simulink model "SIMULACION_RHONN_EFK"  (R2017b)
settings: Solver=VariableStepAuto  StartTime=0.0  StopTime=120  RelTol=1e-3
model workspace (MATLAB code in the model file):
  | %VALORES HUERISTICOS SEGUN EL PAPER
  | %NOTA : los valores cuya definicion se encuentre en minuscula
  | %se utiliza para generar de manera dinamica con programacion
  | %la variable final que se utiliza en el programa.
  | %De manera que si llegara a ser necesario solo se modificarian las variables iniciales
  | 
  | %VARIABLES INICIALES ========================================
  | 
  | p1 = 1 * (10^8);
  | p2 = 1 * (10^2);
  | p3 = 1 * (10^8);
  | p4 = 1 * (10^2);
  | p5 = 1 * (10^2);
  | p6 = 1 * (10^2);
  | p7 = 1 * (10^2);
  | 
  | r1 = 1 * (10^4);
  | r2 = 5 * (10^4);
  | r3 = 1 * (10^4);
  | r4 = 1 * (10^1);
  | r5 = 1 * (10^1);
  | r6 = 1 * (10^3);
  | r7 = 1 * (10^3);
  | 
  | q1 = 5 * (10^5);
  | q2 = 5 * (10^5);
  | q3 = 5 * (10^5);
  | q4 = 1 * (10^1);
  | q5 = 1 * (10^1);
  | q6 = 1 * (10^3);
  | q7 = 1 * (10^3);
  | 
  | G1 = 0.00001;
  | G2 = 0.00001;
  | 
  | %VALOREES INICIALES DE LOS PESOS USADOS EN EKF
  | 
  | %PESOS DE W1
  | W11 = 0.1;
  | W12 = 0.1;
  | %PESOS DE W2
  | W21 = 0.1;
  | W22 = 0.1;
  | %PESOS DE W3
  | W31 = 0.1;
  | W32 = 0.1;
  | %PESOS DE W4
  | W41 = 0.1;
  | W42 = 0.1;
  | W43 = 0.1;
  | W44 = 0.1;
  | %PESOS DE W5
  | W51 = 0.1;
  | W52 = 0.1;
  | W53 = 0.1;
  | W54 = 0.1;
  | %PESOS DE W6
  | W61 = 0.1;
  | W62 = 0.1;
  | W63 = 0.1;
  | W64 = 0.1;
  | %PESOS DE W7
  | W71 = 0.1;
  | W72 = 0.1;
  | W73 = 0.1;
  | W74 = 0.1;
  | 
  | %VALOR DE LAS SIGMOIDALES SUAVES
  | B = 2 * exp(-3);    %Este valor debe ser mayor a cero pero en base a mis observaciones menor a 1.
  | FO = 0.83;   %Este valor es obtenido de la tesis de la Dra Alma debe ser CERCANO y MENOR a 1, si este se vuelve 1 funcionara como FKE unicamente
  | 
  | 
  | %VARIABLES FINALES ========================================
  | 
  | %PARAMETROS DE ENTRENAMIENTO EKF PARA RHONN 1
  | W1 = [W11; W12]; %VALOR INICIAL de Vector de pesos para x1
  | P1 = diag([p1, p1]); %VALOR INICIAL de Matriz diagonal inicial de P1
  | R1 = r1; % Valor de R1
  | Q1 = diag([q1, q1]); % Valor de Q1
  | 
  | %PARAMETROS DE ENTRENAMIENTO EKF PARA RHONN 2
  | W2 = [W21; W22]; %VALOR INICIAL de Vector de pesos para x2
  | P2 = diag([p2, p2]); %VALOR INICIAL de Matriz diagonal inicial de P2
  | R2 = r2; % Valor de R2
  | Q2 = diag([q2, q2]); % Valor de Q2
  | 
  | %PARAMETROS DE ENTRENAMIENTO EKF PARA RHONN 3
  | W3 = [W31; W32]; %VALOR INICIAL de Vector de pesos para x3
  | P3 = diag([p3, p3]); %VALOR INICIAL de Matriz diagonal inicial de P3
  | R3 = r3; % Valor de R3
  | Q3 = diag([q3, q3]); % Valor de Q3
  | 
  | %PARAMETROS DE ENTRENAMIENTO EKF PARA RHONN 4
  | W4 = [W41; W42; W43; W44]; %VALOR INICIAL de Vector de pesos para x4
  | P4 = diag([p4, p4, p4, p4]); %VALOR INICIAL de Matriz diagonal inicial de P4
  | R4 = r4; % Valor de R4
  | Q4 = diag([q4, q4, q4, q4]); % Valor de Q4
  | 
  | %PARAMETROS DE ENTRENAMIENTO EKF PARA RHONN 5
  | W5 = [W51; W52; W53; W54]; %VALOR INICIAL de Vector de pesos para x5
  | P5 = diag([p5, p5, p5, p5]); %VALOR INICIAL de Matriz diagonal inicial de P5
  | R5 = r5; % Valor de R5
  | Q5 = diag([q5, q5, q5, q5]); % Valor de Q5
  | 
  | %PARAMETROS DE ENTRENAMIENTO EKF PARA RHONN 6
  | W6 = [W61; W62; W63; W64]; %VALOR INICIAL de Vector de pesos para x6
  | P6 = diag([p6, p6, p6, p6]); %VALOR INICIAL de Matriz diagonal inicial de P6
  | R6 = r6; % Valor de R6
  | Q6 = diag([q6, q6, q6, q6]); % Valor de Q6
  | 
  | %PARAMETROS DE ENTRENAMIENTO EKF PARA RHONN 7
  | W7 = [W71; W72; W73; W74]; %VALOR INICIAL de Vector de pesos para x7
  | P7 = diag([p7, p7, p7, p7]); %VALOR INICIAL de Matriz diagonal inicial de P7
  | R7 = r7; % Valor de R7
  | Q7 = diag([q7, q7, q7, q7]); % Valor de Q7
libraries: simulink x5
(part 1 of 2)
settings Model: Creator=52324  LastModifiedBy=52324

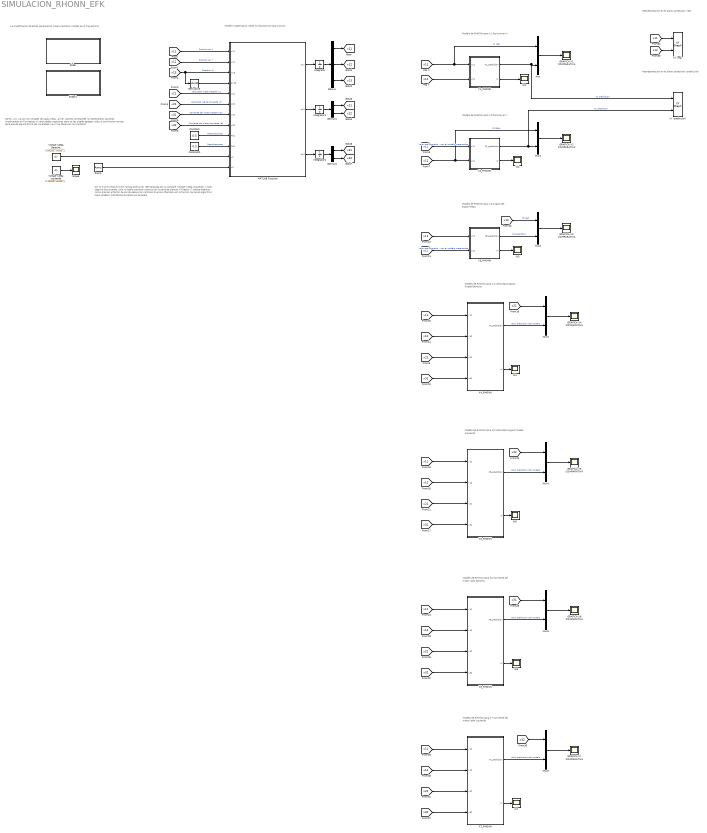
== system SIMULACION_RHONN_EFK ==
  note: por lo mismo esta funcion rampa podria ser reemplazada por la variable 'Voltaje rueda Izquierda'
      | y todo seguira funcionando, solo no habra cambios notorios en la serie de tiempo X4 hasta x7
      |
      | notese ademas como gracias al factor de olvido pese a los cambios bruscos ofrecidos por la funcion rampa
      | el algoritmo logra predecir satisfactoriamente sus estados.
  note: NOTA:
      | u1 y u2 son los voltajes de cada rueda ,
      | al ser valores constantes no representan cambios
      | importantes en Corriestes ni velocidades angulares
      | pero se les puede agregar ruido, o una funcion rampa
      | para que de alguna forma las varaiables x4-x7 se observen con cambios
  note: Representacion en el plano cartesiano 'real'
  note: La modificacion de estos parametros causa cambios visibles en la trayectoria
  note: Modelo matematico robot no holonomico tipo uniciclo
  note: Modelo de RHONN para X1
      | Posicion en X
  note: Modelo de RHONN para X2
      | Posicion en Y
  note: Modelo de RHONN para X3
      | Angulo del Robot Theta
  note: Modelo de RHONN para X4
      | Velocidad Angular Rueda Derecha
  note: Modelo de RHONN para X5
      | Velocidad Angular Rueda Izquierda
  note: Modelo de RHONN para X6
      | Corriente del motor lado derecho
  note: Modelo de RHONN para X7
      | Corriente del motor lado izquierdo
  note: Representacion en el plano cartesiano 'prediccion'
  Constant : Constant  Value=0.5
  Constant1 : Constant  Value=0.5
  Demux : Demux  Outputs=3
  Demux1 : Demux  Outputs=2
  Demux3 : Demux  Outputs=2
  Derivative : Derivative
  GRAFICA X1 COMPARATIVA : Scope
  GRAFICA X2 COMPARATIVA : Scope
  GRAFICA X3 COMPARATIVA : Scope
  GRAFICA X4 COMPARATIVA : Scope
  GRAFICA X5 COMPARATIVA : Scope
  GRAFICA X6 COMPARATIVA : Scope
  GRAFICA X7 COMPARATIVA : Scope
  Integrator : Integrator  InitialCondition=0.1
  Integrator1 : Integrator  InitialCondition=0.1
  Integrator2 : Integrator  InitialCondition=0.1
  MATLAB Function : MATLAB Function  TreatAsAtomicUnit=on
  Mux{,1..6} (7 alike) : Mux  Inputs=2
  Ramp : simulink/Sources/Ramp  slope=0.1  start=0  X0=0
  Scope : Scope
  Slider : Subsystem  DialogController=hmiCreateDDGDialog  IsWebBlock=on  mask(MWDashboardBlock){webBlockId=cf94a416-9279-4ce0-9e8d-8dce151b4ff8, webBlockType=slider, ShowInLibBrowser=on, ShowInitialText=on, HMISrcModelName=SIMULACION_RHONN_EFK}
      mask prompts: webBlockId "WebBlock Id"; webBlockType "WebBlock Type"; HMISrcModelName "Source Model"
      mask help: SimulinkHMI:dialogs:SliderDialogDesc
      mask Help: helpview([docroot '/mapfiles/simulink.map'], 'hmi_slider')
      mask Display:
      | if strcmp(get_param(bdroot(gcb),'BlockDiagramType'), 'library')
      |     image([(matlabroot) '/toolbox/simulink/hmi/icons/Slider.png']);
      | end
  Slider1 : Subsystem  DialogController=hmiCreateDDGDialog  IsWebBlock=on  mask(MWDashboardBlock){webBlockId=98018c70-82f4-44f7-8efb-1d66dbfb8826, webBlockType=slider, ShowInLibBrowser=on, ShowInitialText=on, HMISrcModelName=SIMULACION_RHONN_EFK}
      mask prompts: webBlockId "WebBlock Id"; webBlockType "WebBlock Type"; HMISrcModelName "Source Model"
      mask help: SimulinkHMI:dialogs:SliderDialogDesc
      mask Help: helpview([docroot '/mapfiles/simulink.map'], 'hmi_slider')
      mask Display:
      | if strcmp(get_param(bdroot(gcb),'BlockDiagramType'), 'library')
      |     image([(matlabroot) '/toolbox/simulink/hmi/icons/Slider.png']);
      | end
  Voltaje rueda Derecha : Constant  Value=0.6928571428571
  Voltaje rueda Izquierda : Constant  Value=0.1928571428571
  W{1..7} (7 alike) : Scope
  X1_RHONN : Subsystem
  X2_RHONN : Subsystem
  X3_RHONN : Subsystem
  X4_RHONN : Subsystem
  X5_RHONN : Subsystem
  X6_RHONN : Subsystem
  X7_RHONN : Subsystem
  XY 'prediccion' : simulink/Sinks/XY Graph  xmin=-2.5  xmax=2.5  ymin=-2.5  ymax=2.5  st=-1
  XY 'real' : simulink/Sinks/XY Graph  xmin=-2.5  xmax=2.5  ymin=-2.5  ymax=2.5  st=-1
  tag scope: x11=global, x12=global, x13=global, x21=global, x22=global, x31=global, x32=global
  wires:
  [x11] -> MATLAB Function/1(x11)  "Posicion en X"
  [x12] -> MATLAB Function/2(x12)  "Posicion en Y"
  MATLAB Function/1(dx1) -> Integrator/1
  [x13] -> Derivative/1, MATLAB Function/3(x13)  "Rotacion W"
  Derivative/1 -> MATLAB Function/4(dx13)
  Integrator/1 -> Demux/1
  Demux/3 -> [x13]
  Demux/2 -> [x12]
  MATLAB Function/2(dx2) -> Integrator1/1
  MATLAB Function/3(dx3) -> Integrator2/1
  Integrator1/1 -> Demux1/1
  Integrator2/1 -> Demux3/1
  [x21] -> MATLAB Function/5(x21)  "Velocidad rueda derecha V1"
  [x22] -> MATLAB Function/6(x22)  "Velocidad rueda izquierda V2"
  [x32] -> MATLAB Function/8(x32)  "Corriente del motor izquierdo Ia2"
  Demux1/1 -> [x21]
  Demux1/2 -> [x22]
  Demux3/1 -> [x31]
  Demux3/2 -> [x32]
  Constant/1 -> MATLAB Function/9(Td1)  "Perturbaciones"
  Constant1/1 -> MATLAB Function/10(Td2)  "Perturbaciones"
  X1_RHONN/1(X1_prediction) -> XY 'prediccion'/1, Mux/2  "X1 prediccion"
  Mux/1 -> GRAFICA X1 COMPARATIVA/1
  [x12] -> X1_RHONN/2(x12)
  [x11] -> Mux/1, X1_RHONN/1(x11)  "X1 real"
  [x12] -> Mux1/1, X2_RHONN/2(x12)  "X2 REAL"
  Mux1/1 -> GRAFICA X2 COMPARATIVA/1
  [x11] -> X2_RHONN/1(x11)  "Valor real arrojado por el modelo matematico"
  X2_RHONN/1(X2_prediction) -> XY 'prediccion'/2, Mux1/2  "X2 prediccion"
  [x11] -> X3_RHONN/1(x11)
  [x12] -> X3_RHONN/2(x12)  "Valor real arrojado por el modelo matematico"
  Mux2/1 -> GRAFICA X3 COMPARATIVA/1
  X3_RHONN/1(X3_prediction) -> Mux2/2  "X3 prediccion"
  [x21] -> Mux3/1
  Mux3/1 -> GRAFICA X4 COMPARATIVA/1
  [x12] -> X4_RHONN/2(x12)
  [x11] -> X4_RHONN/1(x11)
  X4_RHONN/1(X4_prediction) -> Mux3/2  "Valor prediccion del modelo"
  [x21] -> X4_RHONN/3(x21)
  [x31] -> X4_RHONN/4(x31)
  [x13] -> Mux2/1  "X3 real"
  [x11] -> X5_RHONN/1(x11)
  X5_RHONN/1(X5_prediction) -> Mux4/2  "Valor prediccion del modelo"
  [x22] -> Mux4/1
  [x12] -> X5_RHONN/2(x12)
  Mux4/1 -> GRAFICA X5 COMPARATIVA/1
  [x21] -> X5_RHONN/3(x21)
  [x31] -> X5_RHONN/4(x31)
  [x31] -> Mux5/1
  [x32] -> X6_RHONN/4(x32)
  [x22] -> X6_RHONN/3(x22)
  Mux5/1 -> GRAFICA X6 COMPARATIVA/1
  [x12] -> X6_RHONN/2(x12)
  X6_RHONN/1(X6_prediction) -> Mux5/2  "Valor prediccion del modelo"
  [x11] -> X6_RHONN/1(x11)
  [x32] -> X7_RHONN/4(x32)
  [x11] -> X7_RHONN/1(x11)
  Mux6/1 -> GRAFICA X7 COMPARATIVA/1
  [x22] -> X7_RHONN/3(x22)
  [x12] -> X7_RHONN/2(x12)
  X7_RHONN/1(X7_prediction) -> Mux6/2  "Valor prediccion del modelo"
  [x32] -> Mux6/1
  X1_RHONN/2(W) -> W1/1
  Demux/1 -> [x11]
  X2_RHONN/2(W) -> W2/1
  X3_RHONN/2(W) -> W3/1
  X4_RHONN/2(W) -> W4/1
  X5_RHONN/2(W) -> W5/1
  X6_RHONN/2(W) -> W6/1
  X7_RHONN/2(W) -> W7/1
  [x31] -> MATLAB Function/7(x31)  "Corriente del motor derecho Ia1"
  [x11] -> XY 'real'/1
  [x12] -> XY 'real'/2
  Voltaje rueda Derecha/1 -> MATLAB Function/11(u1)
  Ramp/1 -> MATLAB Function/12(u2)
  Voltaje rueda Izquierda/1 -> Scope/1

== system SIMULACION_RHONN_EFK/Slider ==

== system SIMULACION_RHONN_EFK/Slider1 ==

== system SIMULACION_RHONN_EFK/X1_RHONN ==
  note: Filtro extendido de kalman (EKF)
  note: Funcion RHONN
      |
      | X(k+1) = w11 * S(x11) + w12 * S(x12)
  x11 : Inport
  x12 : Inport  Port=2
  Generador de matriz H : MATLAB Function  TreatAsAtomicUnit=on
  Sigmoidal suave1 : Subsystem
  Sigmoidal suave3 : Subsystem
  X1_EKF : Subsystem
  X1_RHONN : MATLAB Function  TreatAsAtomicUnit=on
  X1_prediction : Outport
  W : Outport  Port=2
  wires:
  X1_RHONN/1(pred) -> X1_EKF/2(prediccion), X1_prediction/1  "Valor predicho por la red neuronal"
  Sigmoidal suave3/1(salida) -> Generador de matriz H/2(Sx12), X1_RHONN/3(Sx12)  "S(x12)"
  x12/1 -> Sigmoidal suave3/1(c)
  x11/1 -> X1_EKF/1(medicion), Sigmoidal suave1/1(c)
  Sigmoidal suave1/1(salida) -> Generador de matriz H/1(Sx11), X1_RHONN/2(Sx11)  "S(x11)"
  Generador de matriz H/1(H) -> X1_EKF/3(H)  "Valor de matriz H"
  X1_EKF/1(W) -> W/1, X1_RHONN/1(W)  "Valor actualizado de los pesos"

== system SIMULACION_RHONN_EFK/X2_RHONN ==
  note: Filtro extendido de kalman (EKF)
  note: Funcion RHONN
      |
      | X2(k+1) = w21 * S(x11) + w22 * S(x12)
  x11 : Inport
  x12 : Inport  Port=2
  Generador de matriz H : MATLAB Function  TreatAsAtomicUnit=on
  Sigmoidal suave1 : Subsystem
  Sigmoidal suave3 : Subsystem
  X2_EKF : Subsystem
  X2_RHONN_function : MATLAB Function  TreatAsAtomicUnit=on
  X2_prediction : Outport
  W : Outport  Port=2
  wires:
  X2_RHONN_function/1(pred) -> X2_EKF/2(prediccion), X2_prediction/1  "Valor predicho por la red neuronal"
  Sigmoidal suave3/1(salida) -> Generador de matriz H/2(Sx12), X2_RHONN_function/3(Sx12)  "S(x12)"
  x12/1 -> X2_EKF/1(medicion), Sigmoidal suave3/1(c)
  x11/1 -> Sigmoidal suave1/1(c)
  Sigmoidal suave1/1(salida) -> Generador de matriz H/1(Sx11), X2_RHONN_function/2(Sx11)  "S(x11)"
  Generador de matriz H/1(H) -> X2_EKF/3(H)  "Valor de matriz H"
  X2_EKF/1(W) -> X2_RHONN_function/1(W), W/1  "Valor actualizado de los pesos"

== system SIMULACION_RHONN_EFK/X3_RHONN ==
  note: Para este caso el error debe ser basado a la medicion del angulo del robot (x13)
  note: Filtro extendido de kalman (EKF)
  note: Funcion RHONN
      |
      | X3(k+1) = w31 * S(x11) + w32 * S(x12)
  x11 : Inport
  x12 : Inport  Port=2
  Generador de matriz H : MATLAB Function  TreatAsAtomicUnit=on
  Sigmoidal suave1 : Subsystem
  Sigmoidal suave3 : Subsystem
  X3_EKF : Subsystem
  X3_RHONN_function : MATLAB Function  TreatAsAtomicUnit=on
  X3_prediction : Outport
  W : Outport  Port=2
  wires:
  X3_RHONN_function/1(pred) -> X3_EKF/2(prediccion), X3_prediction/1  "Valor predicho por la red neuronal"
  Sigmoidal suave3/1(salida) -> Generador de matriz H/2(Sx12), X3_RHONN_function/3(Sx12)  "S(x12)"
  x12/1 -> Sigmoidal suave3/1(c)
  x11/1 -> Sigmoidal suave1/1(c)
  Sigmoidal suave1/1(salida) -> Generador de matriz H/1(Sx11), X3_RHONN_function/2(Sx11)  "S(x11)"
  Generador de matriz H/1(H) -> X3_EKF/3(H)  "Valor de matriz H"
  X3_EKF/1(W) -> W/1, X3_RHONN_function/1(W)  "Valor actualizado de los pesos"
  [x13] -> X3_EKF/1(medicion)  "Angulo del robot medido"

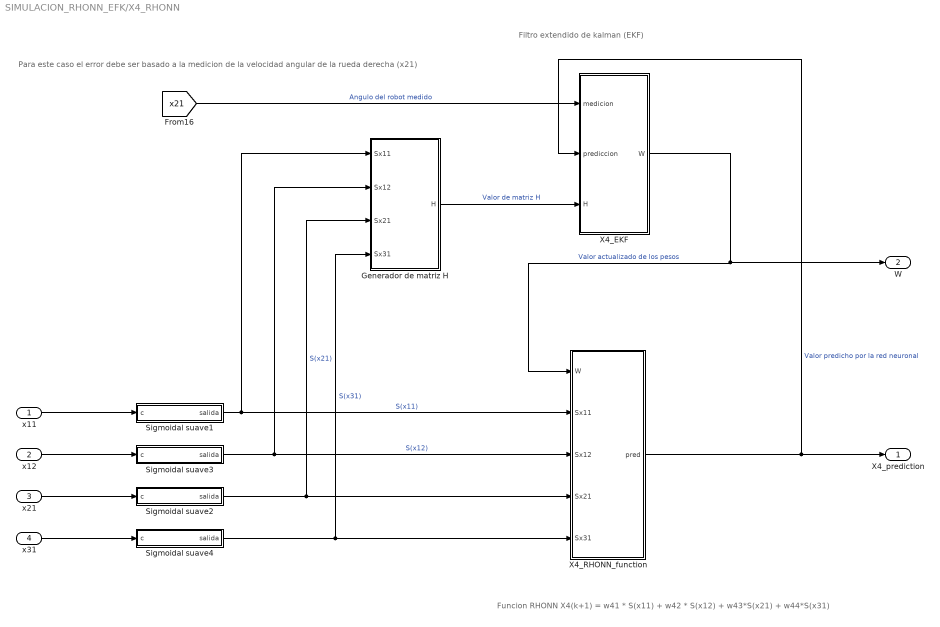
== system SIMULACION_RHONN_EFK/X4_RHONN ==
  note: Para este caso el error debe ser basado a la medicion de la velocidad angular de la rueda derecha (x21)
  note: Filtro extendido de kalman (EKF)
  note: Funcion RHONN
      |
      | X4(k+1) = w41 * S(x11) + w42 * S(x12) + w43*S(x21) + w44*S(x31)
  x11 : Inport
  x12 : Inport  Port=2
  x21 : Inport  Port=3
  x31 : Inport  Port=4
  Generador de matriz H : MATLAB Function  TreatAsAtomicUnit=on
  Sigmoidal suave1 : Subsystem
  Sigmoidal suave2 : Subsystem
  Sigmoidal suave3 : Subsystem
  Sigmoidal suave4 : Subsystem
  X4_EKF : Subsystem
  X4_RHONN_function : MATLAB Function  TreatAsAtomicUnit=on
  X4_prediction : Outport
  W : Outport  Port=2
  wires:
  X4_RHONN_function/1(pred) -> X4_EKF/2(prediccion), X4_prediction/1  "Valor predicho por la red neuronal"
  Sigmoidal suave3/1(salida) -> Generador de matriz H/2(Sx12), X4_RHONN_function/3(Sx12)  "S(x12)"
  x12/1 -> Sigmoidal suave3/1(c)
  x11/1 -> Sigmoidal suave1/1(c)
  Sigmoidal suave1/1(salida) -> Generador de matriz H/1(Sx11), X4_RHONN_function/2(Sx11)  "S(x11)"
  Generador de matriz H/1(H) -> X4_EKF/3(H)  "Valor de matriz H"
  X4_EKF/1(W) -> X4_RHONN_function/1(W), W/1  "Valor actualizado de los pesos"
  [x21] -> X4_EKF/1(medicion)  "Angulo del robot medido"
  x21/1 -> Sigmoidal suave2/1(c)
  x31/1 -> Sigmoidal suave4/1(c)
  Sigmoidal suave2/1(salida) -> Generador de matriz H/3(Sx21), X4_RHONN_function/4(Sx21)  "S(x21)"
  Sigmoidal suave4/1(salida) -> Generador de matriz H/4(Sx31), X4_RHONN_function/5(Sx31)  "S(x31)"

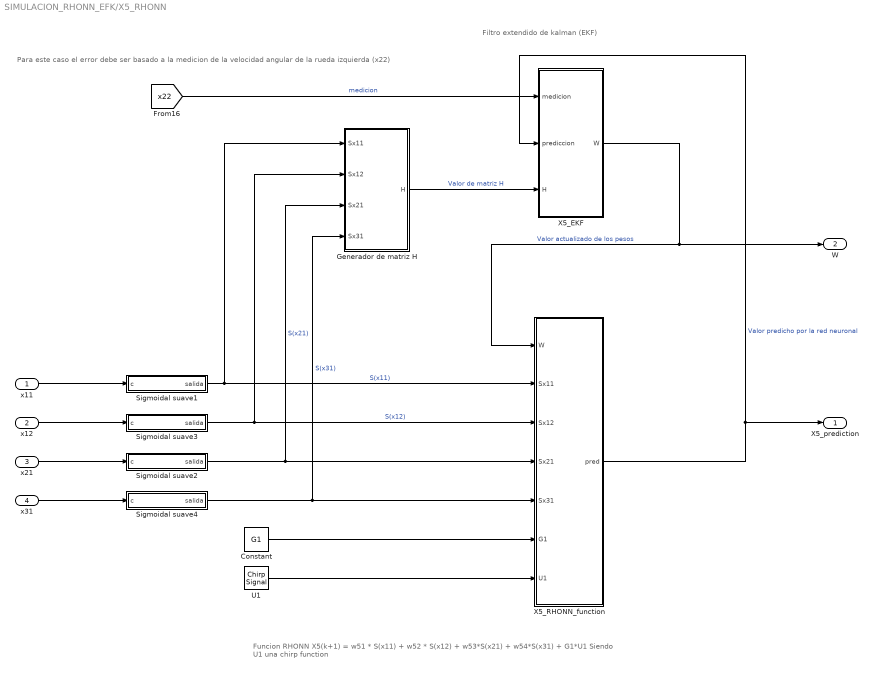
== system SIMULACION_RHONN_EFK/X5_RHONN ==
  note: Para este caso el error debe ser basado a la medicion de la velocidad angular de la rueda izquierda (x22)
  note: Filtro extendido de kalman (EKF)
  note: Funcion RHONN
      |
      | X5(k+1) = w51 * S(x11) + w52 * S(x12) + w53*S(x21) + w54*S(x31) + G1*U1
      |
      | Siendo U1 una chirp function
  x11 : Inport
  x12 : Inport  Port=2
  x21 : Inport  Port=3
  x31 : Inport  Port=4
  Constant : Constant  Value=G1
  Generador de matriz H : MATLAB Function  TreatAsAtomicUnit=on
  Sigmoidal suave1 : Subsystem
  Sigmoidal suave2 : Subsystem
  Sigmoidal suave3 : Subsystem
  Sigmoidal suave4 : Subsystem
  U1 : simulink/Sources/Chirp Signal  f1=0.1  T=100  f2=1
  X5_EKF : Subsystem
  X5_RHONN_function : MATLAB Function  TreatAsAtomicUnit=on
  X5_prediction : Outport
  W : Outport  Port=2
  wires:
  X5_RHONN_function/1(pred) -> X5_EKF/2(prediccion), X5_prediction/1  "Valor predicho por la red neuronal"
  Sigmoidal suave3/1(salida) -> Generador de matriz H/2(Sx12), X5_RHONN_function/3(Sx12)  "S(x12)"
  x12/1 -> Sigmoidal suave3/1(c)
  x11/1 -> Sigmoidal suave1/1(c)
  Sigmoidal suave1/1(salida) -> Generador de matriz H/1(Sx11), X5_RHONN_function/2(Sx11)  "S(x11)"
  Generador de matriz H/1(H) -> X5_EKF/3(H)  "Valor de matriz H"
  X5_EKF/1(W) -> W/1, X5_RHONN_function/1(W)  "Valor actualizado de los pesos"
  [x22] -> X5_EKF/1(medicion)  "medicion"
  x21/1 -> Sigmoidal suave2/1(c)
  x31/1 -> Sigmoidal suave4/1(c)
  Sigmoidal suave2/1(salida) -> Generador de matriz H/3(Sx21), X5_RHONN_function/4(Sx21)  "S(x21)"
  Sigmoidal suave4/1(salida) -> Generador de matriz H/4(Sx31), X5_RHONN_function/5(Sx31)  "S(x31)"
  Constant/1 -> X5_RHONN_function/6(G1)
  U1/1 -> X5_RHONN_function/7(U1)

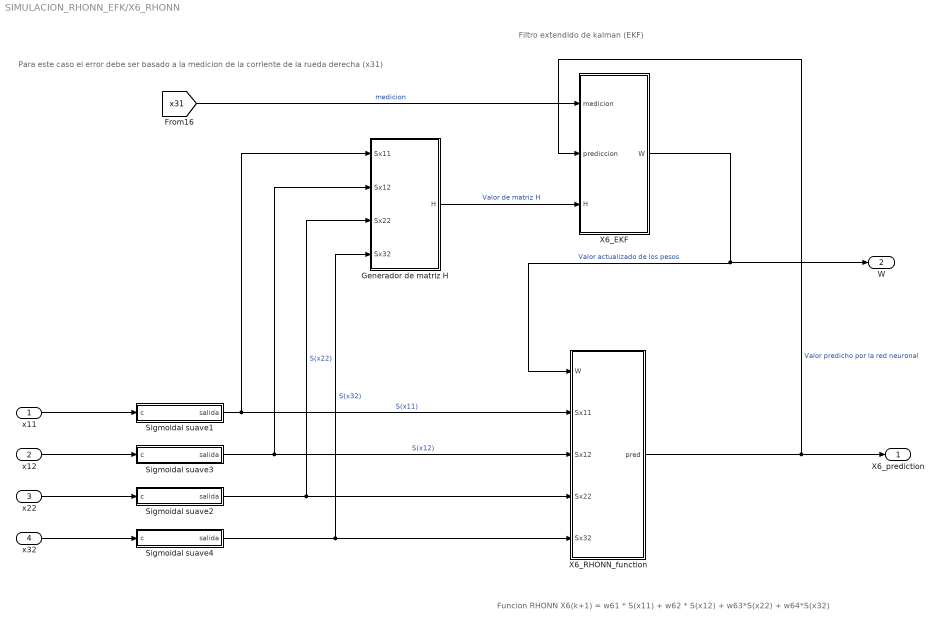
== system SIMULACION_RHONN_EFK/X6_RHONN ==
  note: Para este caso el error debe ser basado a la medicion de la corriente de la rueda derecha (x31)
  note: Filtro extendido de kalman (EKF)
  note: Funcion RHONN
      |
      | X6(k+1) = w61 * S(x11) + w62 * S(x12) + w63*S(x22) + w64*S(x32)
  x11 : Inport
  x12 : Inport  Port=2
  x22 : Inport  Port=3
  x32 : Inport  Port=4
  Generador de matriz H : MATLAB Function  TreatAsAtomicUnit=on
  Sigmoidal suave1 : Subsystem
  Sigmoidal suave2 : Subsystem
  Sigmoidal suave3 : Subsystem
  Sigmoidal suave4 : Subsystem
  X6_EKF : Subsystem
  X6_RHONN_function : MATLAB Function  TreatAsAtomicUnit=on
  X6_prediction : Outport
  W : Outport  Port=2
  wires:
  X6_RHONN_function/1(pred) -> X6_EKF/2(prediccion), X6_prediction/1  "Valor predicho por la red neuronal"
  Sigmoidal suave3/1(salida) -> Generador de matriz H/2(Sx12), X6_RHONN_function/3(Sx12)  "S(x12)"
  x12/1 -> Sigmoidal suave3/1(c)
  x11/1 -> Sigmoidal suave1/1(c)
  Sigmoidal suave1/1(salida) -> Generador de matriz H/1(Sx11), X6_RHONN_function/2(Sx11)  "S(x11)"
  Generador de matriz H/1(H) -> X6_EKF/3(H)  "Valor de matriz H"
  X6_EKF/1(W) -> W/1, X6_RHONN_function/1(W)  "Valor actualizado de los pesos"
  [x31] -> X6_EKF/1(medicion)  "medicion"
  x22/1 -> Sigmoidal suave2/1(c)
  x32/1 -> Sigmoidal suave4/1(c)
  Sigmoidal suave2/1(salida) -> Generador de matriz H/3(Sx22), X6_RHONN_function/4(Sx22)  "S(x22)"
  Sigmoidal suave4/1(salida) -> Generador de matriz H/4(Sx32), X6_RHONN_function/5(Sx32)  "S(x32)"

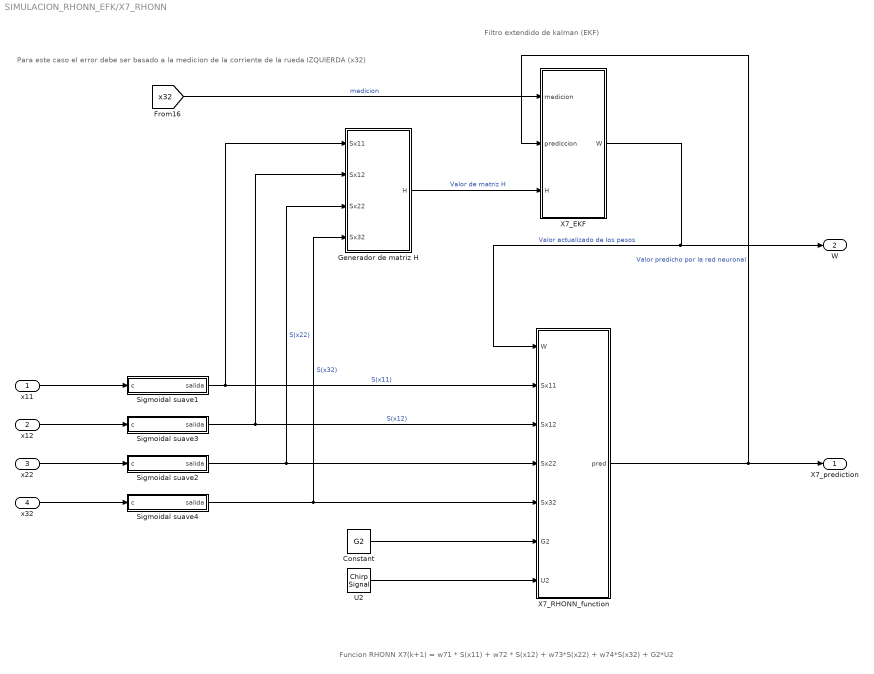
== system SIMULACION_RHONN_EFK/X7_RHONN ==
  note: Para este caso el error debe ser basado a la medicion de la corriente de la rueda IZQUIERDA (x32)
  note: Filtro extendido de kalman (EKF)
  note: Funcion RHONN
      |
      | X7(k+1) = w71 * S(x11) + w72 * S(x12) + w73*S(x22) + w74*S(x32) + G2*U2
  x11 : Inport
  x12 : Inport  Port=2
  x22 : Inport  Port=3
  x32 : Inport  Port=4
  Constant : Constant  Value=G2
  Generador de matriz H : MATLAB Function  TreatAsAtomicUnit=on
  Sigmoidal suave1 : Subsystem
  Sigmoidal suave2 : Subsystem
  Sigmoidal suave3 : Subsystem
  Sigmoidal suave4 : Subsystem
  U2 : simulink/Sources/Chirp Signal  f1=0.1  T=100  f2=1
  X7_EKF : Subsystem
  X7_RHONN_function : MATLAB Function  TreatAsAtomicUnit=on
  X7_prediction : Outport
  W : Outport  Port=2
  wires:
  X7_RHONN_function/1(pred) -> X7_EKF/2(prediccion), X7_prediction/1  "Valor predicho por la red neuronal"
  Sigmoidal suave3/1(salida) -> Generador de matriz H/2(Sx12), X7_RHONN_function/3(Sx12)  "S(x12)"
  x12/1 -> Sigmoidal suave3/1(c)
  x11/1 -> Sigmoidal suave1/1(c)
  Sigmoidal suave1/1(salida) -> Generador de matriz H/1(Sx11), X7_RHONN_function/2(Sx11)  "S(x11)"
  Generador de matriz H/1(H) -> X7_EKF/3(H)  "Valor de matriz H"
  X7_EKF/1(W) -> W/1, X7_RHONN_function/1(W)  "Valor actualizado de los pesos"
  [x32] -> X7_EKF/1(medicion)  "medicion"
  x22/1 -> Sigmoidal suave2/1(c)
  x32/1 -> Sigmoidal suave4/1(c)
  Sigmoidal suave2/1(salida) -> Generador de matriz H/3(Sx22), X7_RHONN_function/4(Sx22)  "S(x22)"
  Sigmoidal suave4/1(salida) -> Generador de matriz H/4(Sx32), X7_RHONN_function/5(Sx32)  "S(x32)"
  Constant/1 -> X7_RHONN_function/6(G2)
  U2/1 -> X7_RHONN_function/7(U2)

== system SIMULACION_RHONN_EFK/X1_RHONN/Sigmoidal suave1 ==
  note: Funcion sigmoidal suave S(*)
  note: Dada la ecuacion (5) del paper:
      | B > 0
      |
      | Y observado en la tesis de la Dra Alma
      | B = 2e^-3
  c : Inport
  Constante de sigmoidal suave : Constant  Value=B
  Sigmoidal suave : MATLAB Function  TreatAsAtomicUnit=on
  salida : Outport
  wires:
  Sigmoidal suave/1(sig) -> salida/1  "Señal transformada S(*)"
  c/1 -> Sigmoidal suave/2(c)  "Señal a transformar"
  Constante de sigmoidal suave/1 -> Sigmoidal suave/1(B)

== system SIMULACION_RHONN_EFK/X1_RHONN/Sigmoidal suave3 ==
  note: Funcion sigmoidal suave S(*)
  note: Dada la ecuacion (5) del paper:
      | B > 0
      |
      | Y observado en la tesis de la Dra Alma
      | B = 2e^-3
  c : Inport
  Constante de sigmoidal suave : Constant  Value=B
  Sigmoidal suave : MATLAB Function  TreatAsAtomicUnit=on
  salida : Outport
  wires:
  Sigmoidal suave/1(sig) -> salida/1  "Señal transformada S(*)"
  c/1 -> Sigmoidal suave/2(c)  "Señal a transformar"
  Constante de sigmoidal suave/1 -> Sigmoidal suave/1(B)

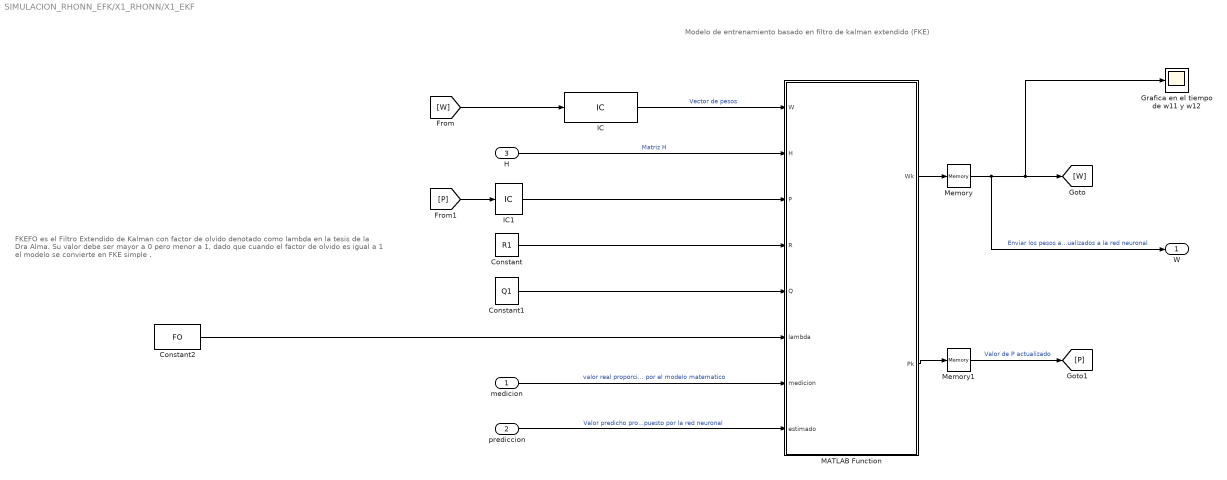
== system SIMULACION_RHONN_EFK/X1_RHONN/X1_EKF ==
  note: FKEFO es el Filtro Extendido de Kalman con factor de olvido
      |
      | denotado como lambda en la tesis de la Dra Alma.
      | Su valor debe ser mayor a 0 pero menor a 1, dado que cuando
      | el factor de olvido es igual a 1 el modelo se convierte en FKE simple .
  note: Modelo de entrenamiento basado en filtro de kalman extendido (FKE)
  medicion : Inport
  prediccion : Inport  Port=2
  H : Inport  Port=3
  Constant : Constant  Value=R1
  Constant1 : Constant  Value=Q1
  Constant2 : Constant  Value=FO
  Grafica en el tiempo de w11 y w12 : Scope
  IC : InitialCondition  Value=W1
  IC1 : InitialCondition  Value=P1
  MATLAB Function : MATLAB Function  TreatAsAtomicUnit=on
  Memory : Memory
  Memory1 : Memory
  W : Outport
  wires:
  prediccion/1 -> MATLAB Function/8(estimado)  "Valor predicho propuesto por la red neuronal"
  medicion/1 -> MATLAB Function/7(medicion)  "valor real proporcionado por el modelo matematico"
  MATLAB Function/1(Wk) -> Memory/1
  [W] -> IC/1
  IC/1 -> MATLAB Function/1(W)  "Vector de pesos"
  MATLAB Function/2(Pk) -> Memory1/1
  IC1/1 -> MATLAB Function/3(P)
  [P] -> IC1/1
  Constant/1 -> MATLAB Function/4(R)
  Constant1/1 -> MATLAB Function/5(Q)
  H/1 -> MATLAB Function/2(H)  "Matriz H"
  Memory1/1 -> [P]  "Valor de P actualizado"
  Memory/1 -> Grafica en el tiempo de w11 y w12/1, [W], W/1  "Enviar los pesos actualizados a la red neuronal"
  Constant2/1 -> MATLAB Function/6(lambda)

== system SIMULACION_RHONN_EFK/X2_RHONN/Sigmoidal suave1 ==
  note: Funcion sigmoidal suave S(*)
  note: Dada la ecuacion (5) del paper:
      | B > 0
      |
      | Y observado en la tesis de la Dra Alma
      | B = 2e^-3
  c : Inport
  Constante de sigmoidal suave : Constant  Value=B
  Sigmoidal suave : MATLAB Function  TreatAsAtomicUnit=on
  salida : Outport
  wires:
  Sigmoidal suave/1(sig) -> salida/1  "Señal transformada S(*)"
  c/1 -> Sigmoidal suave/2(c)  "Señal a transformar"
  Constante de sigmoidal suave/1 -> Sigmoidal suave/1(B)

== system SIMULACION_RHONN_EFK/X2_RHONN/Sigmoidal suave3 ==
  note: Funcion sigmoidal suave S(*)
  note: Dada la ecuacion (5) del paper:
      | B > 0
      |
      | Y observado en la tesis de la Dra Alma
      | B = 2e^-3
  c : Inport
  Constante de sigmoidal suave : Constant  Value=B
  Sigmoidal suave : MATLAB Function  TreatAsAtomicUnit=on
  salida : Outport
  wires:
  Sigmoidal suave/1(sig) -> salida/1  "Señal transformada S(*)"
  c/1 -> Sigmoidal suave/2(c)  "Señal a transformar"
  Constante de sigmoidal suave/1 -> Sigmoidal suave/1(B)

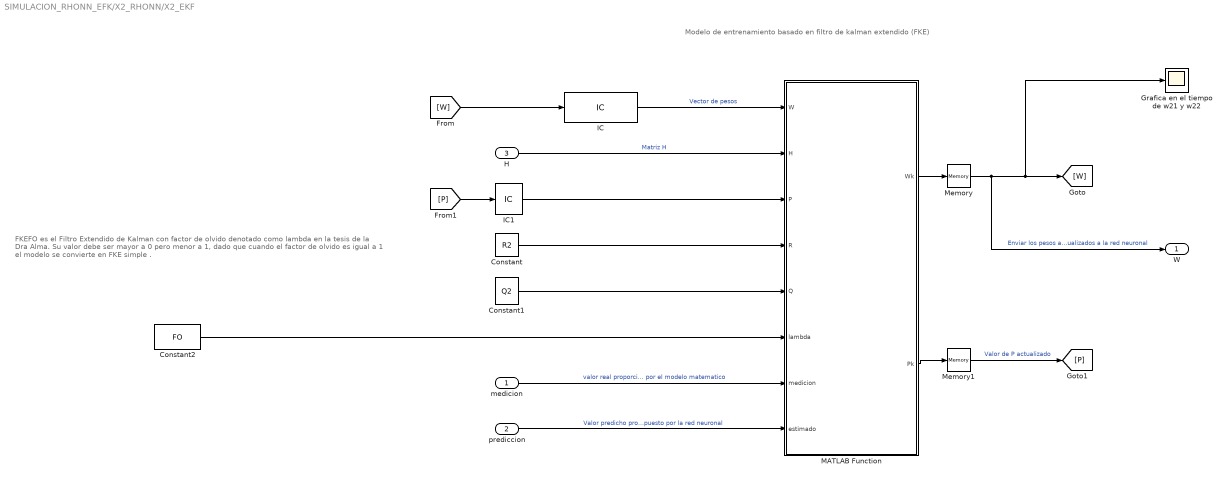
== system SIMULACION_RHONN_EFK/X2_RHONN/X2_EKF ==
  note: FKEFO es el Filtro Extendido de Kalman con factor de olvido
      |
      | denotado como lambda en la tesis de la Dra Alma.
      | Su valor debe ser mayor a 0 pero menor a 1, dado que cuando
      | el factor de olvido es igual a 1 el modelo se convierte en FKE simple .
  note: Modelo de entrenamiento basado en filtro de kalman extendido (FKE)
  medicion : Inport
  prediccion : Inport  Port=2
  H : Inport  Port=3
  Constant : Constant  Value=R2
  Constant1 : Constant  Value=Q2
  Constant2 : Constant  Value=FO
  Grafica en el tiempo de w21 y w22 : Scope
  IC : InitialCondition  Value=W2
  IC1 : InitialCondition  Value=P2
  MATLAB Function : MATLAB Function  TreatAsAtomicUnit=on
  Memory : Memory
  Memory1 : Memory
  W : Outport
  wires:
  prediccion/1 -> MATLAB Function/8(estimado)  "Valor predicho propuesto por la red neuronal"
  medicion/1 -> MATLAB Function/7(medicion)  "valor real proporcionado por el modelo matematico"
  MATLAB Function/1(Wk) -> Memory/1
  [W] -> IC/1
  IC/1 -> MATLAB Function/1(W)  "Vector de pesos"
  MATLAB Function/2(Pk) -> Memory1/1
  IC1/1 -> MATLAB Function/3(P)
  [P] -> IC1/1
  Constant/1 -> MATLAB Function/4(R)
  Constant1/1 -> MATLAB Function/5(Q)
  H/1 -> MATLAB Function/2(H)  "Matriz H"
  Memory1/1 -> [P]  "Valor de P actualizado"
  Memory/1 -> Grafica en el tiempo de w21 y w22/1, [W], W/1  "Enviar los pesos actualizados a la red neuronal"
  Constant2/1 -> MATLAB Function/6(lambda)

== system SIMULACION_RHONN_EFK/X3_RHONN/Sigmoidal suave1 ==
  note: Funcion sigmoidal suave S(*)
  note: Dada la ecuacion (5) del paper:
      | B > 0
      |
      | Y observado en la tesis de la Dra Alma
      | B = 2e^-3
  c : Inport
  Constante de sigmoidal suave : Constant  Value=B
  Sigmoidal suave : MATLAB Function  TreatAsAtomicUnit=on
  salida : Outport
  wires:
  Sigmoidal suave/1(sig) -> salida/1  "Señal transformada S(*)"
  c/1 -> Sigmoidal suave/2(c)  "Señal a transformar"
  Constante de sigmoidal suave/1 -> Sigmoidal suave/1(B)

== system SIMULACION_RHONN_EFK/X3_RHONN/Sigmoidal suave3 ==
  note: Funcion sigmoidal suave S(*)
  note: Dada la ecuacion (5) del paper:
      | B > 0
      |
      | Y observado en la tesis de la Dra Alma
      | B = 2e^-3
  c : Inport
  Constante de sigmoidal suave : Constant  Value=B
  Sigmoidal suave : MATLAB Function  TreatAsAtomicUnit=on
  salida : Outport
  wires:
  Sigmoidal suave/1(sig) -> salida/1  "Señal transformada S(*)"
  c/1 -> Sigmoidal suave/2(c)  "Señal a transformar"
  Constante de sigmoidal suave/1 -> Sigmoidal suave/1(B)

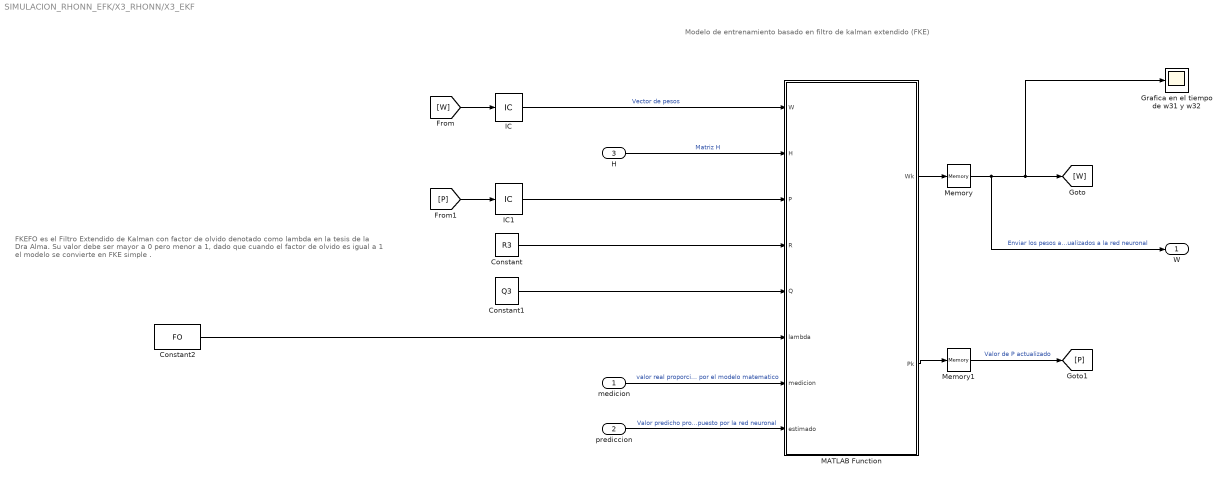
== system SIMULACION_RHONN_EFK/X3_RHONN/X3_EKF ==
  note: FKEFO es el Filtro Extendido de Kalman con factor de olvido
      |
      | denotado como lambda en la tesis de la Dra Alma.
      | Su valor debe ser mayor a 0 pero menor a 1, dado que cuando
      | el factor de olvido es igual a 1 el modelo se convierte en FKE simple .
  note: Modelo de entrenamiento basado en filtro de kalman extendido (FKE)
  medicion : Inport
  prediccion : Inport  Port=2
  H : Inport  Port=3
  Constant : Constant  Value=R3
  Constant1 : Constant  Value=Q3
  Constant2 : Constant  Value=FO
  Grafica en el tiempo de w31 y w32 : Scope
  IC : InitialCondition  Value=W3
  IC1 : InitialCondition  Value=P3
  MATLAB Function : MATLAB Function  TreatAsAtomicUnit=on
  Memory : Memory
  Memory1 : Memory
  W : Outport
  wires:
  prediccion/1 -> MATLAB Function/8(estimado)  "Valor predicho propuesto por la red neuronal"
  medicion/1 -> MATLAB Function/7(medicion)  "valor real proporcionado por el modelo matematico"
  MATLAB Function/1(Wk) -> Memory/1
  [W] -> IC/1
  IC/1 -> MATLAB Function/1(W)  "Vector de pesos"
  MATLAB Function/2(Pk) -> Memory1/1
  IC1/1 -> MATLAB Function/3(P)
  [P] -> IC1/1
  Constant/1 -> MATLAB Function/4(R)
  Constant1/1 -> MATLAB Function/5(Q)
  H/1 -> MATLAB Function/2(H)  "Matriz H"
  Memory1/1 -> [P]  "Valor de P actualizado"
  Memory/1 -> Grafica en el tiempo de w31 y w32/1, [W], W/1  "Enviar los pesos actualizados a la red neuronal"
  Constant2/1 -> MATLAB Function/6(lambda)

== system SIMULACION_RHONN_EFK/X4_RHONN/Sigmoidal suave1 ==
  note: Funcion sigmoidal suave S(*)
  note: Dada la ecuacion (5) del paper:
      | B > 0
      |
      | Y observado en la tesis de la Dra Alma
      | B = 2e^-3
  c : Inport
  Constante de sigmoidal suave : Constant  Value=B
  Sigmoidal suave : MATLAB Function  TreatAsAtomicUnit=on
  salida : Outport
  wires:
  Sigmoidal suave/1(sig) -> salida/1  "Señal transformada S(*)"
  c/1 -> Sigmoidal suave/2(c)  "Señal a transformar"
  Constante de sigmoidal suave/1 -> Sigmoidal suave/1(B)

== system SIMULACION_RHONN_EFK/X4_RHONN/Sigmoidal suave2 ==
  note: Funcion sigmoidal suave S(*)
  note: Dada la ecuacion (5) del paper:
      | B > 0
      |
      | Y observado en la tesis de la Dra Alma
      | B = 2e^-3
  c : Inport
  Constante de sigmoidal suave : Constant  Value=B
  Sigmoidal suave : MATLAB Function  TreatAsAtomicUnit=on
  salida : Outport
  wires:
  Sigmoidal suave/1(sig) -> salida/1  "Señal transformada S(*)"
  c/1 -> Sigmoidal suave/2(c)  "Señal a transformar"
  Constante de sigmoidal suave/1 -> Sigmoidal suave/1(B)

== system SIMULACION_RHONN_EFK/X4_RHONN/Sigmoidal suave3 ==
  note: Funcion sigmoidal suave S(*)
  note: Dada la ecuacion (5) del paper:
      | B > 0
      |
      | Y observado en la tesis de la Dra Alma
      | B = 2e^-3
  c : Inport
  Constante de sigmoidal suave : Constant  Value=B
  Sigmoidal suave : MATLAB Function  TreatAsAtomicUnit=on
  salida : Outport
  wires:
  Sigmoidal suave/1(sig) -> salida/1  "Señal transformada S(*)"
  c/1 -> Sigmoidal suave/2(c)  "Señal a transformar"
  Constante de sigmoidal suave/1 -> Sigmoidal suave/1(B)

== system SIMULACION_RHONN_EFK/X4_RHONN/Sigmoidal suave4 ==
  note: Funcion sigmoidal suave S(*)
  note: Dada la ecuacion (5) del paper:
      | B > 0
      |
      | Y observado en la tesis de la Dra Alma
      | B = 2e^-3
  c : Inport
  Constante de sigmoidal suave : Constant  Value=B
  Sigmoidal suave : MATLAB Function  TreatAsAtomicUnit=on
  salida : Outport
  wires:
  Sigmoidal suave/1(sig) -> salida/1  "Señal transformada S(*)"
  c/1 -> Sigmoidal suave/2(c)  "Señal a transformar"
  Constante de sigmoidal suave/1 -> Sigmoidal suave/1(B)

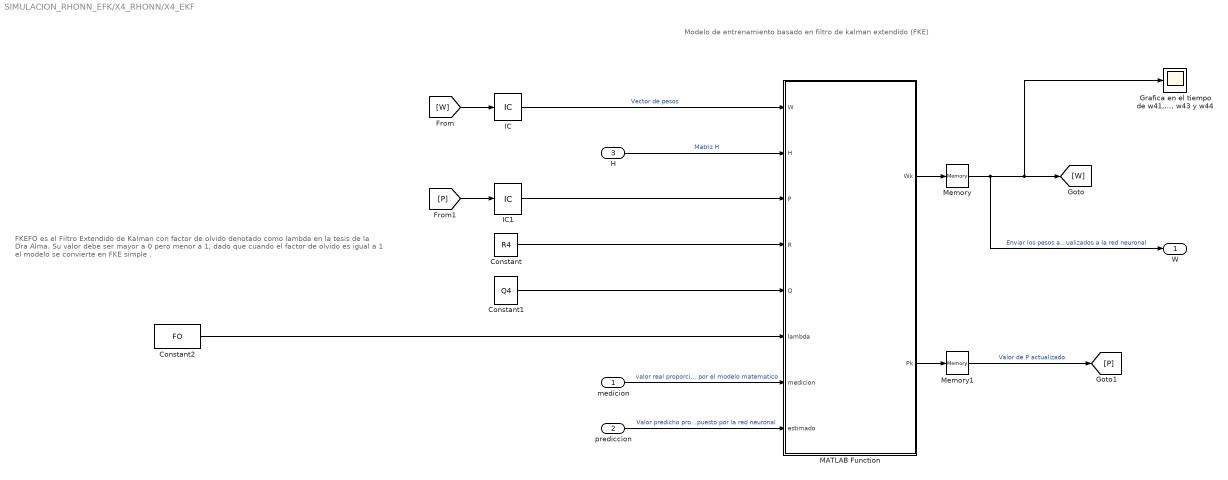
== system SIMULACION_RHONN_EFK/X4_RHONN/X4_EKF ==
  note: FKEFO es el Filtro Extendido de Kalman con factor de olvido
      |
      | denotado como lambda en la tesis de la Dra Alma.
      | Su valor debe ser mayor a 0 pero menor a 1, dado que cuando
      | el factor de olvido es igual a 1 el modelo se convierte en FKE simple .
  note: Modelo de entrenamiento basado en filtro de kalman extendido (FKE)
  medicion : Inport
  prediccion : Inport  Port=2
  H : Inport  Port=3
  Constant : Constant  Value=R4
  Constant1 : Constant  Value=Q4
  Constant2 : Constant  Value=FO
  "Grafica en el tiempo de w41, w42, w43 y w44" : Scope
  IC : InitialCondition  Value=W4
  IC1 : InitialCondition  Value=P4
  MATLAB Function : MATLAB Function  TreatAsAtomicUnit=on
  Memory : Memory
  Memory1 : Memory
  W : Outport
  wires:
  prediccion/1 -> MATLAB Function/8(estimado)  "Valor predicho propuesto por la red neuronal"
  medicion/1 -> MATLAB Function/7(medicion)  "valor real proporcionado por el modelo matematico"
  MATLAB Function/1(Wk) -> Memory/1
  [W] -> IC/1
  IC/1 -> MATLAB Function/1(W)  "Vector de pesos"
  MATLAB Function/2(Pk) -> Memory1/1
  IC1/1 -> MATLAB Function/3(P)
  [P] -> IC1/1
  Constant/1 -> MATLAB Function/4(R)
  Constant1/1 -> MATLAB Function/5(Q)
  H/1 -> MATLAB Function/2(H)  "Matriz H"
  Memory1/1 -> [P]  "Valor de P actualizado"
  Memory/1 -> "Grafica en el tiempo de w41, w42, w43 y w44"/1, [W], W/1  "Enviar los pesos actualizados a la red neuronal"
  Constant2/1 -> MATLAB Function/6(lambda)

== system SIMULACION_RHONN_EFK/X5_RHONN/Sigmoidal suave1 ==
  note: Funcion sigmoidal suave S(*)
  note: Dada la ecuacion (5) del paper:
      | B > 0
      |
      | Y observado en la tesis de la Dra Alma
      | B = 2e^-3
  c : Inport
  Constante de sigmoidal suave : Constant  Value=B
  Sigmoidal suave : MATLAB Function  TreatAsAtomicUnit=on
  salida : Outport
  wires:
  Sigmoidal suave/1(sig) -> salida/1  "Señal transformada S(*)"
  c/1 -> Sigmoidal suave/2(c)  "Señal a transformar"
  Constante de sigmoidal suave/1 -> Sigmoidal suave/1(B)

== system SIMULACION_RHONN_EFK/X5_RHONN/Sigmoidal suave2 ==
  note: Funcion sigmoidal suave S(*)
  note: Dada la ecuacion (5) del paper:
      | B > 0
      |
      | Y observado en la tesis de la Dra Alma
      | B = 2e^-3
  c : Inport
  Constante de sigmoidal suave : Constant  Value=B
  Sigmoidal suave : MATLAB Function  TreatAsAtomicUnit=on
  salida : Outport
  wires:
  Sigmoidal suave/1(sig) -> salida/1  "Señal transformada S(*)"
  c/1 -> Sigmoidal suave/2(c)  "Señal a transformar"
  Constante de sigmoidal suave/1 -> Sigmoidal suave/1(B)

== system SIMULACION_RHONN_EFK/X5_RHONN/Sigmoidal suave3 ==
  note: Funcion sigmoidal suave S(*)
  note: Dada la ecuacion (5) del paper:
      | B > 0
      |
      | Y observado en la tesis de la Dra Alma
      | B = 2e^-3
  c : Inport
  Constante de sigmoidal suave : Constant  Value=B
  Sigmoidal suave : MATLAB Function  TreatAsAtomicUnit=on
  salida : Outport
  wires:
  Sigmoidal suave/1(sig) -> salida/1  "Señal transformada S(*)"
  c/1 -> Sigmoidal suave/2(c)  "Señal a transformar"
  Constante de sigmoidal suave/1 -> Sigmoidal suave/1(B)

== system SIMULACION_RHONN_EFK/X5_RHONN/Sigmoidal suave4 ==
  note: Funcion sigmoidal suave S(*)
  note: Dada la ecuacion (5) del paper:
      | B > 0
      |
      | Y observado en la tesis de la Dra Alma
      | B = 2e^-3
  c : Inport
  Constante de sigmoidal suave : Constant  Value=B
  Sigmoidal suave : MATLAB Function  TreatAsAtomicUnit=on
  salida : Outport
  wires:
  Sigmoidal suave/1(sig) -> salida/1  "Señal transformada S(*)"
  c/1 -> Sigmoidal suave/2(c)  "Señal a transformar"
  Constante de sigmoidal suave/1 -> Sigmoidal suave/1(B)

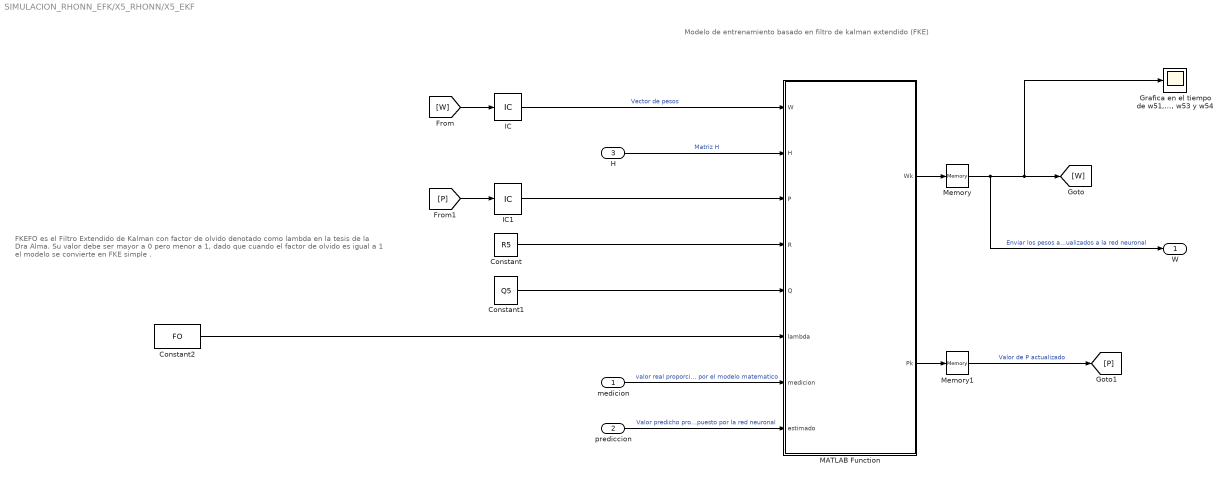
== system SIMULACION_RHONN_EFK/X5_RHONN/X5_EKF ==
  note: FKEFO es el Filtro Extendido de Kalman con factor de olvido
      |
      | denotado como lambda en la tesis de la Dra Alma.
      | Su valor debe ser mayor a 0 pero menor a 1, dado que cuando
      | el factor de olvido es igual a 1 el modelo se convierte en FKE simple .
  note: Modelo de entrenamiento basado en filtro de kalman extendido (FKE)
  medicion : Inport
  prediccion : Inport  Port=2
  H : Inport  Port=3
  Constant : Constant  Value=R5
  Constant1 : Constant  Value=Q5
  Constant2 : Constant  Value=FO
  "Grafica en el tiempo de w51, w52, w53 y w54" : Scope
  IC : InitialCondition  Value=W5
  IC1 : InitialCondition  Value=P5
  MATLAB Function : MATLAB Function  TreatAsAtomicUnit=on
  Memory : Memory
  Memory1 : Memory
  W : Outport
  wires:
  prediccion/1 -> MATLAB Function/8(estimado)  "Valor predicho propuesto por la red neuronal"
  medicion/1 -> MATLAB Function/7(medicion)  "valor real proporcionado por el modelo matematico"
  MATLAB Function/1(Wk) -> Memory/1
  [W] -> IC/1
  IC/1 -> MATLAB Function/1(W)  "Vector de pesos"
  MATLAB Function/2(Pk) -> Memory1/1
  IC1/1 -> MATLAB Function/3(P)
  [P] -> IC1/1
  Constant/1 -> MATLAB Function/4(R)
  Constant1/1 -> MATLAB Function/5(Q)
  H/1 -> MATLAB Function/2(H)  "Matriz H"
  Memory1/1 -> [P]  "Valor de P actualizado"
  Memory/1 -> "Grafica en el tiempo de w51, w52, w53 y w54"/1, [W], W/1  "Enviar los pesos actualizados a la red neuronal"
  Constant2/1 -> MATLAB Function/6(lambda)

== system SIMULACION_RHONN_EFK/X6_RHONN/Sigmoidal suave1 ==
  note: Funcion sigmoidal suave S(*)
  note: Dada la ecuacion (5) del paper:
      | B > 0
      |
      | Y observado en la tesis de la Dra Alma
      | B = 2e^-3
  c : Inport
  Constante de sigmoidal suave : Constant  Value=B
  Sigmoidal suave : MATLAB Function  TreatAsAtomicUnit=on
  salida : Outport
  wires:
  Sigmoidal suave/1(sig) -> salida/1  "Señal transformada S(*)"
  c/1 -> Sigmoidal suave/2(c)  "Señal a transformar"
  Constante de sigmoidal suave/1 -> Sigmoidal suave/1(B)

== system SIMULACION_RHONN_EFK/X6_RHONN/Sigmoidal suave2 ==
  note: Funcion sigmoidal suave S(*)
  note: Dada la ecuacion (5) del paper:
      | B > 0
      |
      | Y observado en la tesis de la Dra Alma
      | B = 2e^-3
  c : Inport
  Constante de sigmoidal suave : Constant  Value=B
  Sigmoidal suave : MATLAB Function  TreatAsAtomicUnit=on
  salida : Outport
  wires:
  Sigmoidal suave/1(sig) -> salida/1  "Señal transformada S(*)"
  c/1 -> Sigmoidal suave/2(c)  "Señal a transformar"
  Constante de sigmoidal suave/1 -> Sigmoidal suave/1(B)

== system SIMULACION_RHONN_EFK/X6_RHONN/Sigmoidal suave3 ==
  note: Funcion sigmoidal suave S(*)
  note: Dada la ecuacion (5) del paper:
      | B > 0
      |
      | Y observado en la tesis de la Dra Alma
      | B = 2e^-3
  c : Inport
  Constante de sigmoidal suave : Constant  Value=B
  Sigmoidal suave : MATLAB Function  TreatAsAtomicUnit=on
  salida : Outport
  wires:
  Sigmoidal suave/1(sig) -> salida/1  "Señal transformada S(*)"
  c/1 -> Sigmoidal suave/2(c)  "Señal a transformar"
  Constante de sigmoidal suave/1 -> Sigmoidal suave/1(B)

== system SIMULACION_RHONN_EFK/X6_RHONN/Sigmoidal suave4 ==
  note: Funcion sigmoidal suave S(*)
  note: Dada la ecuacion (5) del paper:
      | B > 0
      |
      | Y observado en la tesis de la Dra Alma
      | B = 2e^-3
  c : Inport
  Constante de sigmoidal suave : Constant  Value=B
  Sigmoidal suave : MATLAB Function  TreatAsAtomicUnit=on
  salida : Outport
  wires:
  Sigmoidal suave/1(sig) -> salida/1  "Señal transformada S(*)"
  c/1 -> Sigmoidal suave/2(c)  "Señal a transformar"
  Constante de sigmoidal suave/1 -> Sigmoidal suave/1(B)

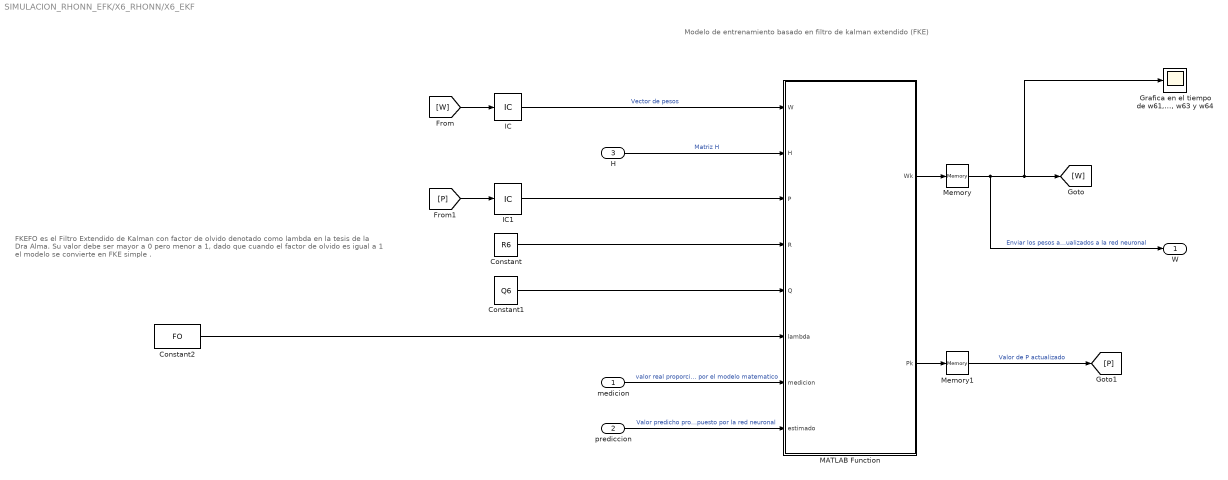
== system SIMULACION_RHONN_EFK/X6_RHONN/X6_EKF ==
  note: FKEFO es el Filtro Extendido de Kalman con factor de olvido
      |
      | denotado como lambda en la tesis de la Dra Alma.
      | Su valor debe ser mayor a 0 pero menor a 1, dado que cuando
      | el factor de olvido es igual a 1 el modelo se convierte en FKE simple .
  note: Modelo de entrenamiento basado en filtro de kalman extendido (FKE)
  medicion : Inport
  prediccion : Inport  Port=2
  H : Inport  Port=3
  Constant : Constant  Value=R6
  Constant1 : Constant  Value=Q6
  Constant2 : Constant  Value=FO
  "Grafica en el tiempo de w61, w62, w63 y w64" : Scope
  IC : InitialCondition  Value=W6
  IC1 : InitialCondition  Value=P6
  MATLAB Function : MATLAB Function  TreatAsAtomicUnit=on
  Memory : Memory
  Memory1 : Memory
  W : Outport
  wires:
  prediccion/1 -> MATLAB Function/8(estimado)  "Valor predicho propuesto por la red neuronal"
  medicion/1 -> MATLAB Function/7(medicion)  "valor real proporcionado por el modelo matematico"
  MATLAB Function/1(Wk) -> Memory/1
  [W] -> IC/1
  IC/1 -> MATLAB Function/1(W)  "Vector de pesos"
  MATLAB Function/2(Pk) -> Memory1/1
  IC1/1 -> MATLAB Function/3(P)
  [P] -> IC1/1
  Constant/1 -> MATLAB Function/4(R)
  Constant1/1 -> MATLAB Function/5(Q)
  H/1 -> MATLAB Function/2(H)  "Matriz H"
  Memory1/1 -> [P]  "Valor de P actualizado"
  Memory/1 -> "Grafica en el tiempo de w61, w62, w63 y w64"/1, [W], W/1  "Enviar los pesos actualizados a la red neuronal"
  Constant2/1 -> MATLAB Function/6(lambda)

== system SIMULACION_RHONN_EFK/X7_RHONN/Sigmoidal suave1 ==
  note: Funcion sigmoidal suave S(*)
  note: Dada la ecuacion (5) del paper:
      | B > 0
      |
      | Y observado en la tesis de la Dra Alma
      | B = 2e^-3
  c : Inport
  Constante de sigmoidal suave : Constant  Value=B
  Sigmoidal suave : MATLAB Function  TreatAsAtomicUnit=on
  salida : Outport
  wires:
  Sigmoidal suave/1(sig) -> salida/1  "Señal transformada S(*)"
  c/1 -> Sigmoidal suave/2(c)  "Señal a transformar"
  Constante de sigmoidal suave/1 -> Sigmoidal suave/1(B)

== system SIMULACION_RHONN_EFK/X7_RHONN/Sigmoidal suave2 ==
  note: Funcion sigmoidal suave S(*)
  note: Dada la ecuacion (5) del paper:
      | B > 0
      |
      | Y observado en la tesis de la Dra Alma
      | B = 2e^-3
  c : Inport
  Constante de sigmoidal suave : Constant  Value=B
  Sigmoidal suave : MATLAB Function  TreatAsAtomicUnit=on
  salida : Outport
  wires:
  Sigmoidal suave/1(sig) -> salida/1  "Señal transformada S(*)"
  c/1 -> Sigmoidal suave/2(c)  "Señal a transformar"
  Constante de sigmoidal suave/1 -> Sigmoidal suave/1(B)

== system SIMULACION_RHONN_EFK/X7_RHONN/Sigmoidal suave3 ==
  note: Funcion sigmoidal suave S(*)
  note: Dada la ecuacion (5) del paper:
      | B > 0
      |
      | Y observado en la tesis de la Dra Alma
      | B = 2e^-3
  c : Inport
  Constante de sigmoidal suave : Constant  Value=B
  Sigmoidal suave : MATLAB Function  TreatAsAtomicUnit=on
  salida : Outport
  wires:
  Sigmoidal suave/1(sig) -> salida/1  "Señal transformada S(*)"
  c/1 -> Sigmoidal suave/2(c)  "Señal a transformar"
  Constante de sigmoidal suave/1 -> Sigmoidal suave/1(B)

== system SIMULACION_RHONN_EFK/X7_RHONN/Sigmoidal suave4 ==
  note: Funcion sigmoidal suave S(*)
  note: Dada la ecuacion (5) del paper:
      | B > 0
      |
      | Y observado en la tesis de la Dra Alma
      | B = 2e^-3
  c : Inport
  Constante de sigmoidal suave : Constant  Value=B
  Sigmoidal suave : MATLAB Function  TreatAsAtomicUnit=on
  salida : Outport
  wires:
  Sigmoidal suave/1(sig) -> salida/1  "Señal transformada S(*)"
  c/1 -> Sigmoidal suave/2(c)  "Señal a transformar"
  Constante de sigmoidal suave/1 -> Sigmoidal suave/1(B)

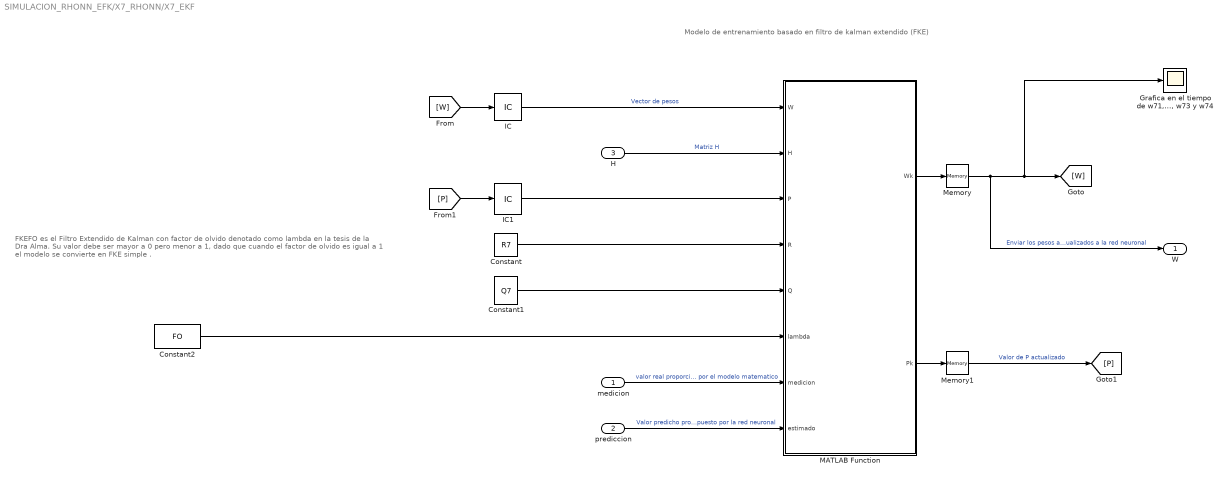
== system SIMULACION_RHONN_EFK/X7_RHONN/X7_EKF ==
  note: FKEFO es el Filtro Extendido de Kalman con factor de olvido
      |
      | denotado como lambda en la tesis de la Dra Alma.
      | Su valor debe ser mayor a 0 pero menor a 1, dado que cuando
      | el factor de olvido es igual a 1 el modelo se convierte en FKE simple .
  note: Modelo de entrenamiento basado en filtro de kalman extendido (FKE)
  medicion : Inport
  prediccion : Inport  Port=2
  H : Inport  Port=3
  Constant : Constant  Value=R7
  Constant1 : Constant  Value=Q7
  Constant2 : Constant  Value=FO
  "Grafica en el tiempo de w71, w72, w73 y w74" : Scope
  IC : InitialCondition  Value=W7
  IC1 : InitialCondition  Value=P7
  MATLAB Function : MATLAB Function  TreatAsAtomicUnit=on
  Memory : Memory
  Memory1 : Memory
  W : Outport
  wires:
  prediccion/1 -> MATLAB Function/8(estimado)  "Valor predicho propuesto por la red neuronal"
  medicion/1 -> MATLAB Function/7(medicion)  "valor real proporcionado por el modelo matematico"
  MATLAB Function/1(Wk) -> Memory/1
  [W] -> IC/1
  IC/1 -> MATLAB Function/1(W)  "Vector de pesos"
  MATLAB Function/2(Pk) -> Memory1/1
  IC1/1 -> MATLAB Function/3(P)
  [P] -> IC1/1
  Constant/1 -> MATLAB Function/4(R)
  Constant1/1 -> MATLAB Function/5(Q)
  H/1 -> MATLAB Function/2(H)  "Matriz H"
  Memory1/1 -> [P]  "Valor de P actualizado"
  Memory/1 -> "Grafica en el tiempo de w71, w72, w73 y w74"/1, [W], W/1  "Enviar los pesos actualizados a la red neuronal"
  Constant2/1 -> MATLAB Function/6(lambda)

== matlab function SIMULACION_RHONN_EFK/X1_RHONN/X1_RHONN ==
  data: W input; pred output; Sx11 input; Sx12 input
function pred = fcn(W,Sx11,Sx12)
    
    %Pesos de la RHONN
    w11 = W(1);
    w12 = W(2);
    %Ecuacion de prediccion
    pred = ( w11 * Sx11 ) + ( w12 * Sx12 );

== matlab function SIMULACION_RHONN_EFK/MATLAB Function ==
  data: x11 input; dx1 output; x12 input; x13 input; dx13 input; x21 input; x22 input; x31 input; x32 input; Td1 input; Td2 input; dx2 output; dx3 output; u1 input; u2 input
function [dx1,dx2,dx3]  = ROBOT(x11, x12, x13, dx13, x21, x22, x31, x32, Td1, Td2, u1, u2)
    
    %Definicion de las matrices de parametros del robot.(Entradas).
    x1 = [x11; x12; x13];
    x2 = [x21; x22];
    x3 = [x31; x32];
    
    %Vector de perturbaciones.
    Td = [Td1; Td2];
    
    %Vector de torques.
    %T = [T1; T2];
   
    %Vector de voltajes
    u = [u1; u2];
    
    %Constantes iniciales
    %La mitad del ancho del robot mobil.
    R = 0.75;
    %La distancia del centro de Pc del robot mobil a la mitad del punto medio
    %de P0 en medio de las ruedas izquierda y derecha.
    d = 0.3;
    %Radio de la rueda.
    r = 0.15;
    %Masa del cuerpo.
    mc = 30;
    %Masa de la rueda con motor.
    mw = 1;
    %Ic,Iw,Im son los momentos de inercia del cuerpo sobre el eje vertical a
    %traves de Pc.
    Ic = 15.625;
    Iw = 0.005;
    Im = 0.0025;
    %Resistencia.
    Ra = diag([2.5,2.5]);
    %Inductancia.
    La = diag([0.048,0.048]);
    %Coeficiente de fuera electromotriz trasero.
    KE = diag([0.02,0.02]);
    %Relacion de transmision.
    N = diag([62.55,62.55]);
    %Constante de torque del motor.
    KT = diag([0.2613,0.2613]);
    %d11, d12 son los coeficientes de amortiguamiento.
    d11 = 0.5;
    d12 = d11;

    %%%%%%%%%%%%%% Constantes productos de otras constantes%%%%%%%%%%%%%%%%%%%%

    %Matriz cinematica del robot
    Jx1 = 0.5*r*[cos(x13), cos(x13); sin(x13), sin(x13); 1/R,-1/R];
    
    m = mc + (2 * mw);
    I = (mc * (d ^ 2)) + (2 * mw * (R^2)) + Ic + (2*Im);
    m11 = 0.25 * ( R ^ -2 ) * (r ^ 2) * ((m * (R ^ 2)) + I) + Iw;
    m12 = 0.25 * ( R ^ -2 ) * (r ^ 2) * ((m * (R ^ 2)) - I);
    M = [m11, m12; m12, m11];
    D = diag([d11, d12]);
    Cdx1 = 0.5 * (1/R) * (r ^ 2) * mc * d * [0, dx13; -dx13 0];
    
    %Definiendo las salidas de la funcion 
    dx1 = Jx1 * x2;
    dx2 = M \( (-Cdx1 * x2) - (D * x2) - Td + (N * KT * x3));
    dx3 = La \ (u - (Ra * x3) - (N * KE * x2));
end

== matlab function SIMULACION_RHONN_EFK/X2_RHONN/Generador de matriz H ==
  data: Sx11 input; H output; Sx12 input
function H = generador_H(Sx11,Sx12)
    %Matrix H para H1 dado 
    %Esta matriz ha sido generada con respecto a la ecuacion 14
    %MAS INFORMACION EN LA OBTENCION DE LA MATRIZ H PARA CADA ESTADO
    % https://github.com/alfredoaguiararce/robot-uniciclo-python/blob/main/Demostracion_de_matrices_H.ipynb
   
    H = [Sx11,Sx12];

== matlab function SIMULACION_RHONN_EFK/X1_RHONN/Sigmoidal suave3/Sigmoidal suave ==
  data: B input; sig output; c input
function sig = fcn(B, c)

%Ecuacion sigmoidal suave
sig = 1/ (1 + exp(-B * c));

== matlab function SIMULACION_RHONN_EFK/X2_RHONN/Sigmoidal suave1/Sigmoidal suave ==
  data: B input; sig output; c input
function sig = fcn(B, c)

%Ecuacion sigmoidal suave
sig = 1/ (1 + exp(-B * c));

== matlab function SIMULACION_RHONN_EFK/X1_RHONN/Sigmoidal suave1/Sigmoidal suave ==
  data: B input; sig output; c input
function sig = fcn(B, c)

%Ecuacion sigmoidal suave
sig = 1/ (1 + exp(-B * c));

== matlab function SIMULACION_RHONN_EFK/X1_RHONN/X1_EKF/MATLAB Function ==
  data: W input; Wk output; H input; P input; R input; Q input; lambda input; medicion input; estimado input; Pk output
function [Wk,Pk] = fcn(W, H, P, R, Q, lambda, medicion, estimado)

    % NOTA: Para este caso
    % W, H, P, R, Q representan los valores en k_esima
    % Wk, Pk representan los valores de k + 1
    
    %L es el numero total de pesos = 2 (w11,w12)
    %m es el numero de salidas = 1 (X(k+1))
    
    %P es una matriz L x L (2x2)
    %R es una matriz m x m (1x1)
    %Q es una matriz L x L (2x2)
    %K es una matriz L x m (2x1)
    
    %lambda es el factor de olvido si lambda = 1 el modelo deja de ser
    %FKEFO y se vuelve FKE
    
    %Mi(k)
    M = (R * lambda ) + (H * P * H');
    %K(k)
    K = (P * H' )/(M);
    %W(k+1)
    Wk = W + K * (medicion - estimado);
    %P(k+1)
    Pk = (P * (1/lambda)) - ((1/lambda) * K * H * P) + Q;

== matlab function SIMULACION_RHONN_EFK/X1_RHONN/Generador de matriz H ==
  data: Sx11 input; H output; Sx12 input
function H = generador_H(Sx11,Sx12)
    %Matrix H para H1 dado 
    %Esta matriz ha sido generada con respecto a la ecuacion 14
    H = [Sx11,Sx12];

== matlab function SIMULACION_RHONN_EFK/X2_RHONN/Sigmoidal suave3/Sigmoidal suave ==
  data: B input; sig output; c input
function sig = fcn(B, c)

%Ecuacion sigmoidal suave
sig = 1/ (1 + exp(-B * c));

== matlab function SIMULACION_RHONN_EFK/X2_RHONN/X2_EKF/MATLAB Function ==
  data: W input; Wk output; H input; P input; R input; Q input; lambda input; medicion input; estimado input; Pk output
function [Wk,Pk] = fcn(W, H, P, R, Q, lambda, medicion, estimado)

    % NOTA: Para este caso
    % W, H, P, R, Q representan los valores en k_esima
    % Wk, Pk representan los valores de k + 1
    
    %L es el numero total de pesos = 2 (w11,w12)
    %m es el numero de salidas = 1 (X(k+1))
    
    %P es una matriz L x L (2x2)
    %R es una matriz m x m (1x1)
    %Q es una matriz L x L (2x2)
    %K es una matriz L x m (2x1)
    
    %lambda es el factor de olvido si lambda = 1 el modelo deja de ser
    %FKEFO y se vuelve FKE
    
    %Mi(k)
    M = (R * lambda ) + (H * P * H');
    %K(k)
    K = (P * H' )/(M);
    %W(k+1)
    Wk = W + K * (medicion - estimado);
    %P(k+1)
    Pk = (P * (1/lambda)) - ((1/lambda) * K * H * P) + Q;

== matlab function SIMULACION_RHONN_EFK/X2_RHONN/X2_RHONN_function ==
  data: W input; pred output; Sx11 input; Sx12 input
function pred = fcn(W,Sx11,Sx12)

    %Pesos de X2
    w21 = W(1);
    w22 = W(2);
    %ecuacion de prediccion X2
    pred = ( w21 * Sx11 ) + ( w22 * Sx12 );

== matlab function SIMULACION_RHONN_EFK/X3_RHONN/Generador de matriz H ==
  data: Sx11 input; H output; Sx12 input
function H = generador_H(Sx11,Sx12)
    %Matrix H para H1 dado 
    %Esta matriz ha sido generada con respecto a la ecuacion 14
    %MAS INFORMACION EN LA OBTENCION DE LA MATRIZ H PARA CADA ESTADO
    % https://github.com/alfredoaguiararce/robot-uniciclo-python/blob/main/Demostracion_de_matrices_H.ipynb
   
    H = [Sx11,Sx12];

== matlab function SIMULACION_RHONN_EFK/X3_RHONN/Sigmoidal suave1/Sigmoidal suave ==
  data: B input; sig output; c input
function sig = fcn(B, c)

%Ecuacion sigmoidal suave
sig = 1/ (1 + exp(-B * c));

== matlab function SIMULACION_RHONN_EFK/X3_RHONN/Sigmoidal suave3/Sigmoidal suave ==
  data: B input; sig output; c input
function sig = fcn(B, c)

%Ecuacion sigmoidal suave
sig = 1/ (1 + exp(-B * c));

== matlab function SIMULACION_RHONN_EFK/X3_RHONN/X3_EKF/MATLAB Function ==
  data: W input; Wk output; H input; P input; R input; Q input; lambda input; medicion input; estimado input; Pk output
function [Wk,Pk] = fcn(W, H, P, R, Q, lambda, medicion, estimado)

    % NOTA: Para este caso
    % W, H, P, R, Q representan los valores en k_esima
    % Wk, Pk representan los valores de k + 1
    
    %L es el numero total de pesos = 2 (w11,w12)
    %m es el numero de salidas = 1 (X(k+1))
    
    %P es una matriz L x L (2x2)
    %R es una matriz m x m (1x1)
    %Q es una matriz L x L (2x2)
    %K es una matriz L x m (2x1)
    
    %lambda es el factor de olvido si lambda = 1 el modelo deja de ser
    %FKEFO y se vuelve FKE
    
    %Mi(k)
    M = (R * lambda ) + (H * P * H');
    %K(k)
    K = (P * H' )/(M);
    %W(k+1)
    Wk = W + K * (medicion - estimado);
    %P(k+1)
    Pk = (P * (1/lambda)) - ((1/lambda) * K * H * P) + Q;

== matlab function SIMULACION_RHONN_EFK/X3_RHONN/X3_RHONN_function ==
  data: W input; pred output; Sx11 input; Sx12 input
function pred = fcn(W,Sx11,Sx12)

    %Pesos de X3
    w31 = W(1);
    w32 = W(2);
    %ecuacion de prediccion X2
    pred = ( w31 * Sx11 ) + ( w32 * Sx12 );

== matlab function SIMULACION_RHONN_EFK/X4_RHONN/Generador de matriz H ==
  data: Sx11 input; H output; Sx12 input; Sx21 input; Sx31 input
function H = generador_H(Sx11,Sx12,Sx21,Sx31)
    %Matrix H para H1 dado 
    %Esta matriz ha sido generada con respecto a la ecuacion 14
    %MAS INFORMACION EN LA OBTENCION DE LA MATRIZ H PARA CADA ESTADO
    % https://github.com/alfredoaguiararce/robot-uniciclo-python/blob/main/Demostracion_de_matrices_H.ipynb
   
    H = [Sx11,Sx12,Sx21,Sx31];

== matlab function SIMULACION_RHONN_EFK/X4_RHONN/Sigmoidal suave1/Sigmoidal suave ==
  data: B input; sig output; c input
function sig = fcn(B, c)

%Ecuacion sigmoidal suave
sig = 1/ (1 + exp(-B * c));

== matlab function SIMULACION_RHONN_EFK/X4_RHONN/Sigmoidal suave3/Sigmoidal suave ==
  data: B input; sig output; c input
function sig = fcn(B, c)

%Ecuacion sigmoidal suave
sig = 1/ (1 + exp(-B * c));
